simulink model "compare_lin_non_lin"  (R2022b)
settings: Solver=FixedStepAuto  StartTime=0.0  StopTime=RunTime  FixedStep=time_step  RelTol=1e-3
values from neighbouring files (symbols this model uses):
  A = [0 0.00936734307998 0 -119.348579139 0 1 -103.40359731 0 -22.3994836329 0 0 -0.229713482044 ... (25 elements, 5x5)]    [System.mat]    (also in linearize_operating_point.m = double(A))
  B = [0 0 0 0 500]    [System.mat]    (also in linearize_operating_point.m = double(B))
  C = [1  0  0  0  0; 0  0  1  0  0]    [System.mat]    (also in linearize_operating_point.m = [1 0 0 0 0)
  D = [0 0]    [System.mat]    (also in linearize_operating_point.m = zeros(2,1))
  T_0 = x_op(5)    [run_compare_lin_non_lin.m]
  theta_1_0 = x_op(1)    [run_compare_lin_non_lin.m]
  theta_2_0 = x_op(3)    [run_compare_lin_non_lin.m]
  theta_d_1_0 = x_op(2)    [run_compare_lin_non_lin.m]
  theta_d_2_0 = x_op(4)    [run_compare_lin_non_lin.m]
  x_op = [0 0 3.14159265359 0 0]    [System.mat]    (also in linearize_operating_point.m = [init_theta_1; 0; init_theta_2; 0; 0])
settings Model: Creator=annel  LastModifiedBy=annel

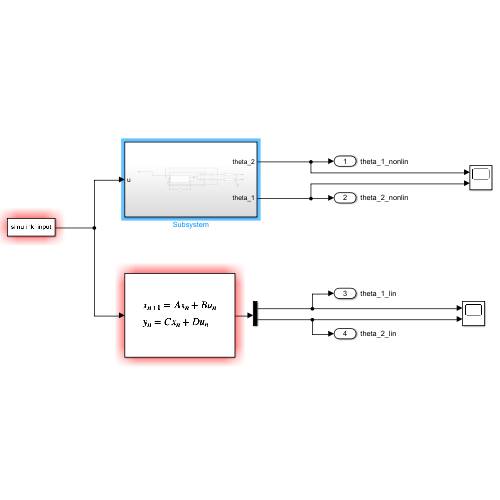
[thumbnail: Simulink's stored preview of the top-level diagram]
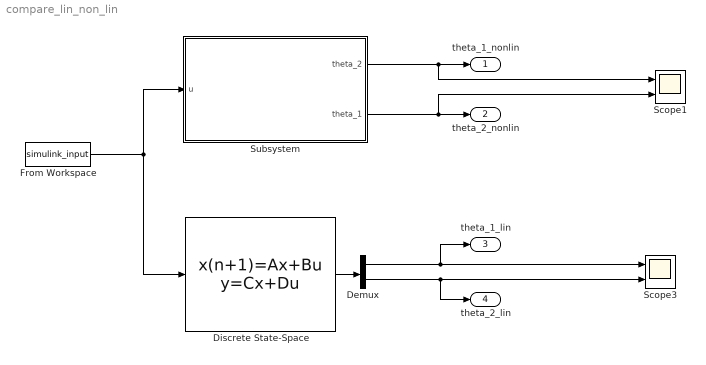
== system compare_lin_non_lin ==
  Demux : Demux  Outputs=2
  Discrete State-Space : DiscreteStateSpace  A=A  B=B  C=C  D=D  InitialCondition=x_op  SampleTime=-1
  From Workspace : FromWorkspace
  Scope1 : Scope  NumInputPorts=2
  Scope3 : Scope  NumInputPorts=2
  Subsystem : Subsystem
  theta_1_nonlin : Outport
  theta_2_nonlin : Outport  Port=2
  theta_1_lin : Outport  Port=3
  theta_2_lin : Outport  Port=4
  wires:
  Subsystem/1(theta_2) -> theta_1_nonlin/1, Scope1/1
  From Workspace/1 -> Discrete State-Space/1, Subsystem/1(u)
  Subsystem/2(theta_1) -> Scope1/2, theta_2_nonlin/1
  Discrete State-Space/1 -> Demux/1
  Demux/1 -> theta_1_lin/1, Scope3/1
  Demux/2 -> theta_2_lin/1, Scope3/2

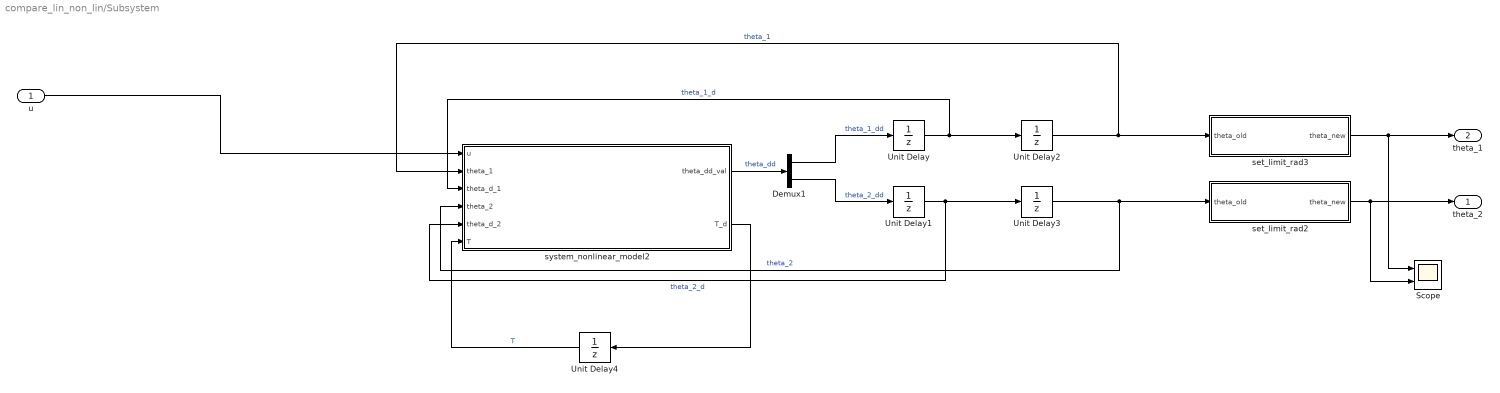
== system compare_lin_non_lin/Subsystem ==
  u : Inport
  Demux1 : Demux  Outputs=2
  Scope : Scope  NumInputPorts=2
  Unit Delay : UnitDelay  InitialCondition=theta_d_1_0  SampleTime=-1  HasFrameUpgradeWarning=on
  Unit Delay1 : UnitDelay  InitialCondition=theta_d_2_0  SampleTime=-1  HasFrameUpgradeWarning=on
  Unit Delay2 : UnitDelay  InitialCondition=theta_1_0  SampleTime=-1  HasFrameUpgradeWarning=on
  Unit Delay3 : UnitDelay  InitialCondition=theta_2_0  SampleTime=-1  HasFrameUpgradeWarning=on
  Unit Delay4 : UnitDelay  InitialCondition=T_0  SampleTime=-1  HasFrameUpgradeWarning=on
  set_limit_rad2 : MATLAB Function  TreatAsAtomicUnit=on
  set_limit_rad3 : MATLAB Function  TreatAsAtomicUnit=on
  system_nonlinear_model2 : MATLAB Function  TreatAsAtomicUnit=on
  theta_2 : Outport
  theta_1 : Outport  Port=2
  wires:
  set_limit_rad3/1(theta_new) -> theta_1/1, Scope/1
  Unit Delay2/1 -> system_nonlinear_model2/2(theta_1), set_limit_rad3/1(theta_old)  "theta_1"
  Unit Delay3/1 -> system_nonlinear_model2/4(theta_2), set_limit_rad2/1(theta_old)  "theta_2"
  u/1 -> system_nonlinear_model2/1(u)
  Unit Delay1/1 -> system_nonlinear_model2/5(theta_d_2), Unit Delay3/1  "theta_2_d"
  set_limit_rad2/1(theta_new) -> theta_2/1, Scope/2
  system_nonlinear_model2/1(theta_dd_val) -> Demux1/1  "theta_dd"
  Demux1/2 -> Unit Delay1/1  "theta_2_dd"
  Demux1/1 -> Unit Delay/1  "theta_1_dd"
  Unit Delay/1 -> system_nonlinear_model2/3(theta_d_1), Unit Delay2/1  "theta_1_d"
  system_nonlinear_model2/2(T_d) -> Unit Delay4/1
  Unit Delay4/1 -> system_nonlinear_model2/6(T)  "T"

== matlab function compare_lin_non_lin/Subsystem/system_nonlinear_model2 ==
  settings: updateMethod=DISCRETE  sampleTime=0.001
  data: u input size=1; theta_dd_val output size=2; T_d output; theta_1 input size=1; theta_d_1 input size=1; theta_2 input size=1; theta_d_2 input size=1; T input; params parameter
function [theta_dd_val, T_d] = get_theta_dt_dt(u, theta_1, theta_d_1, theta_2, theta_d_2, T, params)

k_m_0 = params(7);
tau_e_0 = params(8);

T_d = (1/tau_e_0)*T + (k_m_0/tau_e_0)*u;

% theta_dd_val = NonLinFunc(T,theta_1,theta_2,theta_d_1,theta_d_2); % this
% does not work, because simulink is stupid.

theta_dd_val = [
                                                                                                                                                                   (2177205792337185200000*sin(theta_1 + theta_2)*(7101996468378179*cos(theta_2) + 5837472162125388))/(59390441777463697512*cos(theta_2) + 157619855740175396464645510487628125*cos(theta_2)^2 - 67469767625708245300871903596602750000) - theta_d_2*((1152921504606846976*(7101996468378179*cos(theta_2) + 5837472162125388))/(59390441777463697512*cos(theta_2) + 157619855740175396464645510487628125*cos(theta_2)^2 - 67469767625708245300871903596602750000) + (336507359412909324930676272031334400000*sin(theta_2)*((7101996468378179*theta_d_1)/18446744073709551616 + (7101996468378179*theta_d_2)/18446744073709551616))/(59390441777463697512*cos(theta_2) + 157619855740175396464645510487628125*cos(theta_2)^2 - 67469767625708245300871903596602750000)) - theta_d_1*((336507359412909324930676272031334400000*((7101996468378179*theta_d_2*sin(theta_2))/18446744073709551616 - 5171/250))/(59390441777463697512*cos(theta_2) + 157619855740175396464645510487628125*cos(theta_2)^2 - 67469767625708245300871903596602750000) + (22193738963681809375*theta_d_1*sin(theta_2)*(7101996468378179*cos(theta_2) + 5837472162125388))/(59390441777463697512*cos(theta_2) + 157619855740175396464645510487628125*cos(theta_2)^2 - 67469767625708245300871903596602750000)) - (336507359412909324930676272031334400000*T)/(59390441777463697512*cos(theta_2) + 157619855740175396464645510487628125*cos(theta_2)^2 - 67469767625708245300871903596602750000) - (336507359412909324930676272031334400000*((5443014480842963*sin(theta_1 + theta_2))/144115188075855872 + (3446064362871357*sin(theta_1))/72057594037927936))/(59390441777463697512*cos(theta_2) + 157619855740175396464645510487628125*cos(theta_2)^2 - 67469767625708245300871903596602750000)
theta_d_1*((57646075230342348800000*(7101996468378179*cos(theta_2) + 5837472162125388)*((7101996468378179*theta_d_2*sin(theta_2))/18446744073709551616 - 5171/250))/(59390441777463697512*cos(theta_2) + 157619855740175396464645510487628125*cos(theta_2)^2 - 67469767625708245300871903596602750000) + (7272444383619255296*theta_d_1*sin(theta_2)*(43347146413441024*cos(theta_2) + 11304968154247740625))/(59390441777463697512*cos(theta_2) + 157619855740175396464645510487628125*cos(theta_2)^2 - 67469767625708245300871903596602750000)) + theta_d_2*((1180591620717411303424*(43347146413441024*cos(theta_2) + 11304968154247740625))/(3125*(59390441777463697512*cos(theta_2) + 157619855740175396464645510487628125*cos(theta_2)^2 - 67469767625708245300871903596602750000)) + (57646075230342348800000*sin(theta_2)*(7101996468378179*cos(theta_2) + 5837472162125388)*((7101996468378179*theta_d_1)/18446744073709551616 + (7101996468378179*theta_d_2)/18446744073709551616))/(59390441777463697512*cos(theta_2) + 157619855740175396464645510487628125*cos(theta_2)^2 - 67469767625708245300871903596602750000)) + (57646075230342348800000*T*(7101996468378179*cos(theta_2) + 5837472162125388))/(59390441777463697512*cos(theta_2) + 157619855740175396464645510487628125*cos(theta_2)^2 - 67469767625708245300871903596602750000) + (57646075230342348800000*(7101996468378179*cos(theta_2) + 5837472162125388)*((5443014480842963*sin(theta_1 + theta_2))/144115188075855872 + (3446064362871357*sin(theta_1))/72057594037927936))/(59390441777463697512*cos(theta_2) + 157619855740175396464645510487628125*cos(theta_2)^2 - 67469767625708245300871903596602750000) - (713426794033048846336*sin(theta_1 + theta_2)*(43347146413441024*cos(theta_2) + 11304968154247740625))/(59390441777463697512*cos(theta_2) + 157619855740175396464645510487628125*cos(theta_2)^2 - 67469767625708245300871903596602750000)
];

== matlab function compare_lin_non_lin/Subsystem/set_limit_rad2 ==
  settings: updateMethod=DISCRETE  sampleTime=0.001
  data: theta_old input size=1; theta_new output size=1
function theta_new   = set_limit_rad(theta_old)

theta_new = theta_old - floor(theta_old / 2 / pi) * 2 * pi;
theta_new = theta_old;

== matlab function compare_lin_non_lin/Subsystem/set_limit_rad3 ==
  settings: updateMethod=DISCRETE  sampleTime=0.001
  data: theta_old input size=1; theta_new output size=1
function theta_new   = set_limit_rad(theta_old)

theta_new = theta_old - floor(theta_old / 2 / pi) * 2 * pi;
theta_new = theta_old;
